simulink model "P84s"  (R2015b)
settings: Solver=VariableStepAuto  StartTime=0.0  StopTime=4  RelTol=1e-3
settings Model: Creator=xmax1946  LastModifiedBy=xmax1946

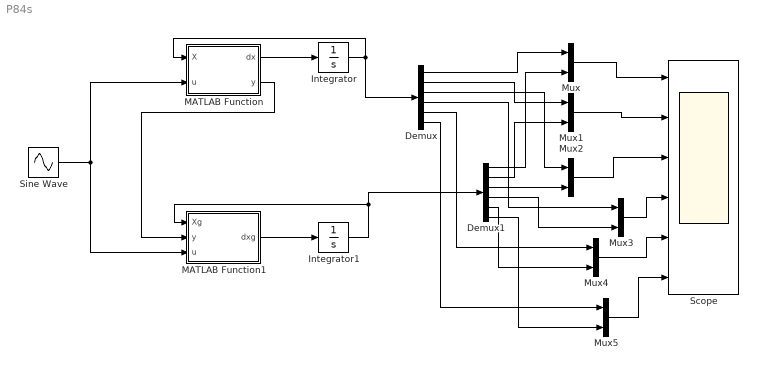
== system P84s ==
  Demux : Demux  Outputs=6
  Demux1 : Demux  Outputs=6
  Integrator : Integrator  InitialCondition=[100;100;100;100;100;100]
  Integrator1 : Integrator  InitialCondition=[1;1;1;1;1;1]
  MATLAB Function : MATLAB Function  TreatAsAtomicUnit=on
  MATLAB Function1 : MATLAB Function  TreatAsAtomicUnit=on
  Mux{,1..5} (6 alike) : Mux  Inputs=2
  Scope : Scope  NumInputPorts=6
  Sine Wave : Sin  Amplitude=10  SampleTime=0
  wires:
  MATLAB Function/1(dx) -> Integrator/1
  MATLAB Function1/1(dxg) -> Integrator1/1
  Integrator/1 -> MATLAB Function/1(X), Demux/1
  MATLAB Function/2(y) -> MATLAB Function1/2(y)
  Integrator1/1 -> Demux1/1, MATLAB Function1/1(Xg)
  Demux/1 -> Mux/1
  Demux1/1 -> Mux/2
  Demux/2 -> Mux1/1
  Demux1/2 -> Mux1/2
  Demux/3 -> Mux2/1
  Demux1/3 -> Mux2/2
  Mux/1 -> Scope/1
  Mux1/1 -> Scope/2
  Mux2/1 -> Scope/3
  Sine Wave/1 -> MATLAB Function1/3(u), MATLAB Function/2(u)
  Mux3/1 -> Scope/4
  Demux/4 -> Mux3/1
  Demux1/4 -> Mux3/2
  Mux4/1 -> Scope/5
  Demux/5 -> Mux4/1
  Demux1/5 -> Mux4/2
  Demux/6 -> Mux5/1
  Demux1/6 -> Mux5/2
  Mux5/1 -> Scope/6

== matlab function P84s/MATLAB Function1 ==
  data: Xg input; y input; u input; dxg output
function dxg =fcn(Xg,y,u)
A=[0,1,0,0,0,0;16,0,-8,0,0,0;0,0,0,1,0,0;-16,0,16,0,0,0;0,0,0,0,0,1;0,0,0,0,0,0];
B=[0;-1;0;0;0;1];
C=[1,0,1,0,1,0];
L=[-369.0625;-1.7052e+03;314.7500;1.9613e+03;80.3125;60.9375];
dxg=A*Xg+B*u+L*(y-C*Xg);

== matlab function P84s/MATLAB Function ==
  data: dx output; X input; y output; u input
function [dx,y]=fcn(X,u)
A=[0,1,0,0,0,0;16,0,-8,0,0,0;0,0,0,1,0,0;-16,0,16,0,0,0;0,0,0,0,0,1;0,0,0,0,0,0];
B=[0;-1;0;0;0;1];
C=[1,0,1,0,1,0];
dx=A*X+B*u;
y=C*X;
